simulink model "quadrotor_model"  (R2024b)
settings: Solver=VariableStepAuto  StartTime=0.0  StopTime=10.0  RelTol=1e-3
values from neighbouring files (symbols this model uses):
  b = 0.001    [exercise_2_simulink.m]    (also in exercise_2_simulink_2.m)
  D = diag([.01 .01 .01])    [exercise_2_simulink.m]    (also in exercise_2_simulink_2.m)
  eul0 = [0 0 0]'    [exercise_2_simulink.m]
  g_i = [0 0 -9.81]'    [exercise_2_simulink.m]    (also in exercise_2_simulink_2.m)
  Ixx = 3e-6    (= 3e-06)    [exercise_2_simulink.m]    (also in exercise_2_simulink_2.m)
  Iyy = 3e-6    (= 3e-06)    [exercise_2_simulink.m]    (also in exercise_2_simulink_2.m)
  Izz = 1e-5    (= 1e-05)    [exercise_2_simulink.m]    (also in exercise_2_simulink_2.m)
  k = 0.01    [exercise_2_simulink.m]    (also in exercise_2_simulink_2.m; uas_parameters.m = 0.0176714586764)
  L = 0.225    [exercise_2_simulink.m]    (also in exercise_2_simulink_2.m)
  m = 0.5    [exercise_2_simulink.m]    (also in exercise_2_simulink_2.m)
  omega = cases{i,2}    [exercise_2_simulink.m]    (also in exercise_2_simulink_2.m)
  p0 = [0 0 0]'    [exercise_2_simulink.m]    (also in exercise_2_simulink_2.m)
  v0 = [0 0 0]'    [exercise_2_simulink.m]    (also in exercise_2_simulink_2.m)
  w0 = [0 0 0]'    [exercise_2_simulink.m]    (also in exercise_2_simulink_2.m)
settings Model: Creator=claes  LastModifiedBy=claes

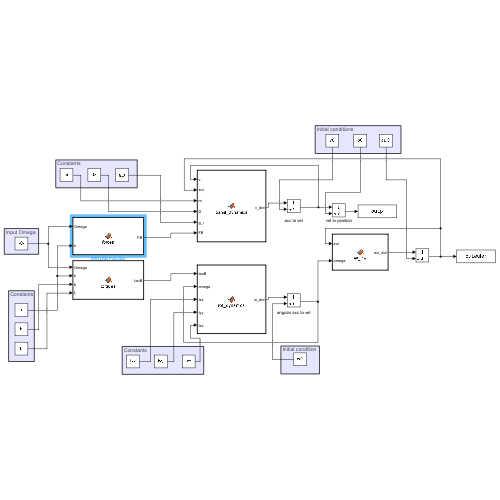
[thumbnail: Simulink's stored preview of the top-level diagram]
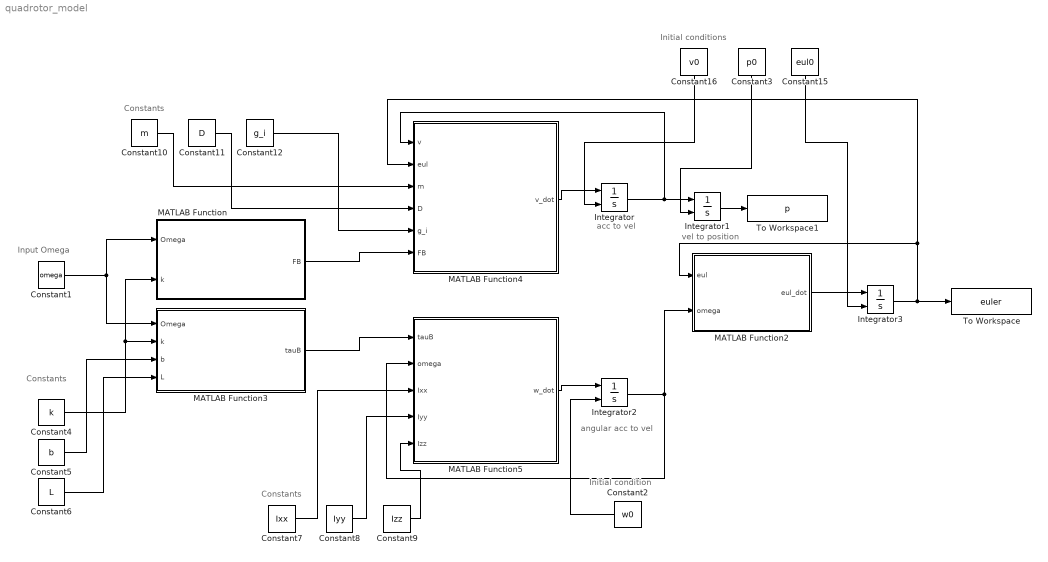
== system quadrotor_model ==
  note: angular acc to vel
  note: Initial condition
  note: Input Omega
  note: Constants
  note: Constants
  note: Constants
  note: Initial conditions
  note: acc to vel
  note: vel to position
  Constant1 : Constant  Value=omega
  Constant10 : Constant  Value=m
  Constant11 : Constant  Value=D
  Constant12 : Constant  Value=g_i
  Constant15 : Constant  Value=eul0
  Constant16 : Constant  Value=v0
  Constant2 : Constant  Value=w0
  Constant3 : Constant  Value=p0
  Constant4 : Constant  Value=k
  Constant5 : Constant  Value=b
  Constant6 : Constant  Value=L
  Constant7 : Constant  Value=Ixx
  Constant8 : Constant  Value=Iyy
  Constant9 : Constant  Value=Izz
  Integrator : Integrator  InitialConditionSource=external
  Integrator1 : Integrator  InitialConditionSource=external
  Integrator2 : Integrator  InitialConditionSource=external  InitialCondition=w0
  Integrator3 : Integrator  InitialConditionSource=external
  MATLAB Function : MATLAB Function  TreatAsAtomicUnit=on
  MATLAB Function2 : MATLAB Function  TreatAsAtomicUnit=on
  MATLAB Function3 : MATLAB Function  TreatAsAtomicUnit=on
  MATLAB Function4 : MATLAB Function  TreatAsAtomicUnit=on
  MATLAB Function5 : MATLAB Function  TreatAsAtomicUnit=on
  To Workspace : ToWorkspace  VariableName=euler  SaveFormat=Timeseries  SampleTime=-1
  To Workspace1 : ToWorkspace  VariableName=p  SaveFormat=Timeseries  SampleTime=-1
  wires:
  Constant4/1 -> MATLAB Function/2(k), MATLAB Function3/2(k)
  Constant1/1 -> MATLAB Function3/1(Omega), MATLAB Function/1(Omega)
  Constant5/1 -> MATLAB Function3/3(b)
  Constant6/1 -> MATLAB Function3/4(L)
  MATLAB Function/1(FB) -> MATLAB Function4/6(FB)
  MATLAB Function3/1(tauB) -> MATLAB Function5/1(tauB)
  Constant7/1 -> MATLAB Function5/3(Ixx)
  Constant8/1 -> MATLAB Function5/4(Iyy)
  Constant9/1 -> MATLAB Function5/5(Izz)
  Constant10/1 -> MATLAB Function4/3(m)
  Constant11/1 -> MATLAB Function4/4(D)
  Constant12/1 -> MATLAB Function4/5(g_i)
  MATLAB Function4/1(v_dot) -> Integrator/1
  MATLAB Function5/1(w_dot) -> Integrator2/1
  Integrator/1 -> MATLAB Function4/1(v), Integrator1/1
  Integrator2/1 -> MATLAB Function2/2(omega), MATLAB Function5/2(omega)
  Constant2/1 -> Integrator2/2
  Integrator1/1 -> To Workspace1/1
  Constant16/1 -> Integrator/2
  Constant15/1 -> Integrator3/2
  MATLAB Function2/1(eul_dot) -> Integrator3/1
  Integrator3/1 -> MATLAB Function2/1(eul), MATLAB Function4/2(eul), To Workspace/1
  Constant3/1 -> Integrator1/2

== matlab function quadrotor_model/MATLAB Function ==
  data: Omega input; FB output; k input
function FB  = forces(Omega, k)
    % omega = [ω1 ω2 ω3 ω4]'  (rad/s)
    T = k*sum(Omega.^2);      % total thrust magnitude
    FB = [0;0;T];             % thrust in body frame (z_b)
end

== matlab function quadrotor_model/MATLAB Function2 ==
  data: eul input; eul_dot output; omega input
function eul_dot = W_inv(eul ,omega)

    phi   = eul(1); % Roll angle
    theta = eul(2); % Pitch angle
    psi   = eul(3); % Yaw angle

    sphi = sin(phi);  cphi = cos(phi);
    tth  = tan(theta); cth = cos(theta);
    W = [ 1  sphi*tth  cphi*tth;
          0     cphi      -sphi;
          0  sphi/cth  cphi/cth ];
    eul_dot = W*omega;
end

== matlab function quadrotor_model/MATLAB Function3 ==
  data: Omega input; tauB output; k input; b input; L input
function tauB  = torques(Omega, k, b, L)
    % omega = [ω1 ω2 ω3 ω4]'  (rad/s)
    tauB = [ L*k*(Omega(1)^2 - Omega(3)^2);     % roll
             L*k*(Omega(2)^2 - Omega(4)^2);     % pitch
             b*(Omega(1)^2 - Omega(2)^2 + Omega(3)^2 - Omega(4)^2) ];
end

== matlab function quadrotor_model/MATLAB Function4 ==
  data: v input; eul input; m input; D input; g_i input; FB input; v_dot output
function v_dot = transl_dynamics(v, eul, m, D, g_i, FB)
% FB      : 3×1    (N)   thrust expressed in the BODY frame
% v       : 3×1    (m/s) inertial linear velocity
% eul_a   : 3x1 (rad)   Euler angles [phi; theta; psi] representing
%                             the orientation of the body-fixed frame w.r.t.
%                             the inertial frame.
%                             phi   : roll angle
%                             theta : pitch angle
%                             psi   : yaw angle
% m       : mass
% D       : 3×3 drag matrix
% g_i     : 3×1 gravity in inertial frame

% Extract individual Euler angles from the input vector
phi   = eul(1); % Roll angle
theta = eul(2); % Pitch angle
psi   = eul(3); % Yaw angle

% 1) body → inertial
cphi = cos(phi); sphi = sin(phi);
cth  = cos(theta); sth  = sin(theta);
cps  = cos(psi); sps = sin(psi);

R11 =  cth*cps;          
R12 =  cth*sps;          
R13 = -sth;
R21 =  sphi*sth*cps - cphi*sps;
R22 =  sphi*sth*sps + cphi*cps;
R23 =  sphi*cth;
R31 =  cphi*sth*cps + sphi*sps;
R32 =  cphi*sth*sps - sphi*cps;
R33 =  cphi*cth;

FB_i = [R11 R12 R13;
        R21 R22 R23;
        R31 R32 R33] * FB;

% 2) drag (already in inertial frame)
FD_i = -D * v;

% 3) Newton
v_dot = (1/m)*( FB_i + FD_i ) + g_i;
end

== matlab function quadrotor_model/MATLAB Function5 ==
  data: tauB input; omega input; w_dot output; Ixx input; Iyy input; Izz input
function w_dot = rot_dynamics(tauB, omega, Ixx, Iyy, Izz)
% tauB : 3×1   (N·m)      body torques
% omega: 3×1   (rad/s)    current body angular velocity

I  = diag([Ixx Iyy Izz]);
invI = diag([1/Ixx 1/Iyy 1/Izz]);

w_cross_Iw = [  0       -omega(3)  omega(2);
                omega(3)  0       -omega(1);
               -omega(2)  omega(1) 0 ] * (I*omega);

w_dot = invI * ( tauB - w_cross_Iw );
end
